simulink model "PID_CARTESIANO"  (R2015a)
settings: Solver=ode45  StartTime=0.0  StopTime=Tfinal  RelTol=1e-3
values from neighbouring files (symbols this model uses):
  Ki1 = 0    [INICIO.m]
  Ki2 = 0    [INICIO.m]
  Ki3 = 0    [INICIO.m]
  Ki4 = 0    [INICIO.m]
  Kp1 = 100    [INICIO.m]
  Kp2 = 100    [INICIO.m]
  Kp3 = 100    [INICIO.m]
  Kp4 = 100    [INICIO.m]
  Kv1 = 10    [INICIO.m]
  Kv2 = 10    [INICIO.m]
  Kv3 = 10    [INICIO.m]
  Kv4 = 10    [INICIO.m]
  Tem = 0.001    [INICIO.m]    (also in circular.m)
undefined symbols (not defined in the file or in its folder): diferencia, mgd, mgi
libraries: simulink x1
settings Model: CovHtmlReporting=off  Creator=ANDRES Y MARCELA  LastModifiedBy=Shadow
settings DataIOCC: SignalLoggingSaveFormat=ModelDataLogs
settings OptimizationCC: ExpressionDepthLimit=2147483647
settings DebuggingCC: UnderspecifiedInitializationDetection=Classic  MergeDetectMultiDrivingBlocksExec=none  SolverPrmCheckMsg=warning  FcnCallInpInsideContextMsg=EnableAllAsWarning  StateNameClashWarn=warning
settings GRTTargetCC: CombineOutputUpdateFcns=off  GRTInterface=on

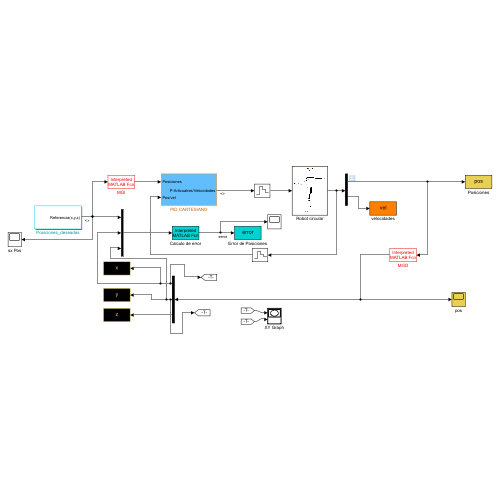
[thumbnail: Simulink's stored preview of the top-level diagram]
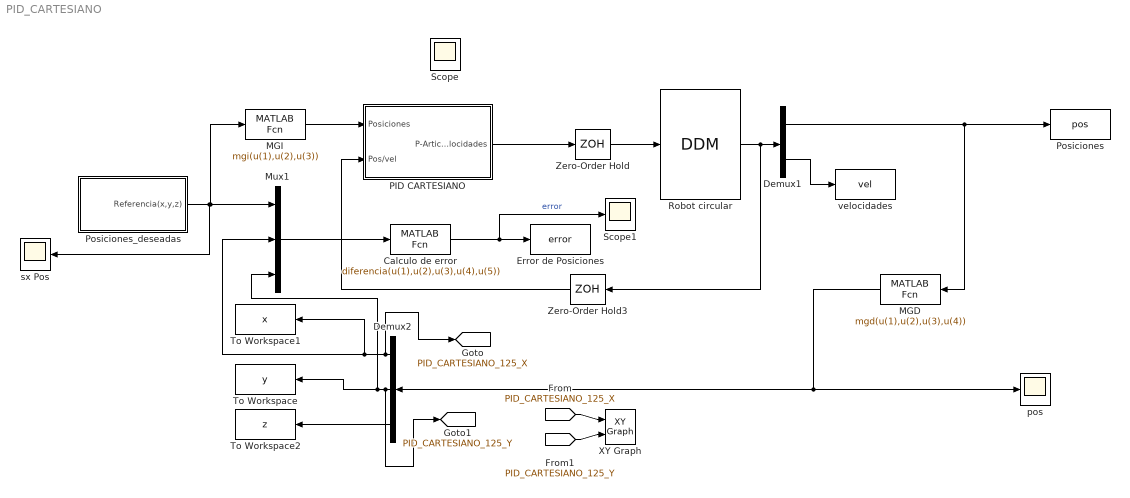
== system PID_CARTESIANO ==
  Calculo de error : MATLABFcn  MATLABFcn=diferencia(u(1),u(2),u(3),u(4),u(5))
  Demux1 : Demux  Outputs=2
  Demux2 : Demux  Outputs=3
  Error de Posiciones : ToWorkspace  VariableName=error  SampleTime=-1
  MGD : MATLABFcn  MATLABFcn=mgd(u(1),u(2),u(3),u(4))
  MGI : MATLABFcn  MATLABFcn=mgi(u(1),u(2),u(3))
  Mux1 : Mux  Inputs=3
  PID CARTESIANO : Subsystem
  Posiciones : ToWorkspace  VariableName=pos  SampleTime=-1
  Posiciones_deseadas : Subsystem
  Robot circular : S-Function  FunctionName=DDM  Parameters=QI  SFunctionDeploymentMode=off  EnableBusSupport=off
      mask Display:
      | %  find_system('Name','robot');
      |  image(imread('robot.jpg'))
  Scope1 : Scope
      settings: TimeRange=auto  MaxDataPoints=5000  SaveToWorkspace=off  SaveName=ScopeData2  YMin=-0.00006  YMax=0.00051  SampleTime=-1
  To Workspace : ToWorkspace  VariableName=y  SampleTime=-1
  To Workspace1 : ToWorkspace  VariableName=x  SampleTime=-1
  To Workspace2 : ToWorkspace  VariableName=z  SampleTime=-1
  XY Graph : simulink/Sinks/XY Graph  xmin=-1  xmax=1  ymin=-1  ymax=1  st=-1
  Zero-Order Hold : ZeroOrderHold  SampleTime=Tem
  Zero-Order Hold3 : ZeroOrderHold  SampleTime=Tem
  pos : Scope
      settings: TimeRange=3  LimitDataPoints=on  MaxDataPoints=5000  SaveToWorkspace=off  SaveName=ScopeData4  YMin=0.36498  YMax=0.51503  SampleTime=-1
  sx Pos : Scope
      settings: TimeRange=3  LimitDataPoints=on  MaxDataPoints=5000  SaveToWorkspace=off  SaveName=ScopeData2  YMin=0.365  YMax=0.515  SampleTime=-1
  velocidades : ToWorkspace  VariableName=vel  SampleTime=-1
  Scope : Scope
      settings: TimeRange=auto  MaxDataPoints=5000  SaveToWorkspace=off  YMin=-1.01882  YMax=0.95883  SampleTime=-1
  tag scope: PID_CARTESIANO_125_X=global, PID_CARTESIANO_125_Y=global
  wires:
  MGI/1 -> PID CARTESIANO/1(Posiciones)
  Demux1/2 -> velocidades/1
  Posiciones_deseadas/1(Referencia(x,y,z)) -> MGI/1, Mux1/1, sx Pos/1
  Demux2/3 -> To Workspace2/1
  Robot circular/1 -> Zero-Order Hold3/1, Demux1/1
  Zero-Order Hold/1 -> Robot circular/1
  Mux1/1 -> Calculo de error/1
  Zero-Order Hold3/1 -> PID CARTESIANO/2(Pos/vel)
  Calculo de error/1 -> Error de Posiciones/1, Scope1/1  "error"
  Demux2/1 -> To Workspace1/1, Mux1/2, [PID_CARTESIANO_125_X]
  Demux2/2 -> To Workspace/1, Mux1/3, [PID_CARTESIANO_125_Y]
  MGD/1 -> pos/1, Demux2/1
  Demux1/1 -> Posiciones/1, MGD/1
  PID CARTESIANO/1(P-Articualres/Velocidades) -> Zero-Order Hold/1
  [PID_CARTESIANO_125_X] -> XY Graph/1
  [PID_CARTESIANO_125_Y] -> XY Graph/2

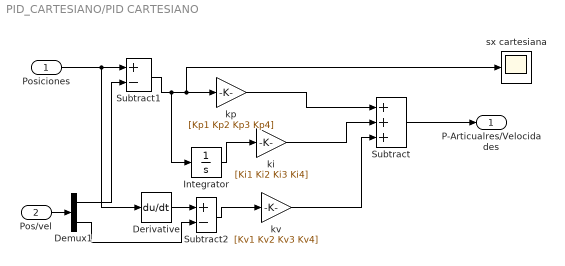
== system PID_CARTESIANO/PID CARTESIANO ==
  Posiciones : Inport
  Pos/vel : Inport  Port=2
  Demux1 : Demux  Outputs=2
  Derivative : Derivative
  Integrator : Integrator
  Subtract : Sum  Inputs=+++
  Subtract1 : Sum  Inputs=+-
  Subtract2 : Sum  Inputs=+-
  ki : Gain  Gain=[Ki1 Ki2 Ki3 Ki4]
  kp : Gain  Gain=[Kp1 Kp2 Kp3 Kp4]
  kv : Gain  Gain=[Kv1 Kv2 Kv3 Kv4]
  sx cartesiana : Scope
      settings: TimeRange=3  LimitDataPoints=on  MaxDataPoints=5000  SaveToWorkspace=off  YMin=-0.00012  YMax=0.00023  SampleTime=-1
  P-Articualres/Velocidades : Outport
  wires:
  Subtract1/1 -> Integrator/1, kp/1, sx cartesiana/1
  Derivative/1 -> Subtract2/1
  Subtract2/1 -> kv/1
  kp/1 -> Subtract/1
  Integrator/1 -> ki/1
  Pos/vel/1 -> Demux1/1
  Posiciones/1 -> Derivative/1, Subtract1/1
  Subtract/1 -> P-Articualres/Velocidades/1
  Demux1/1 -> Subtract1/2
  Demux1/2 -> Subtract2/2
  ki/1 -> Subtract/2
  kv/1 -> Subtract/3

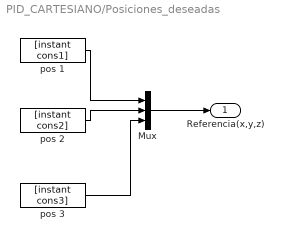
== system PID_CARTESIANO/Posiciones_deseadas ==
  Mux : Mux  Inputs=3
  pos 1 : FromWorkspace  VariableName=[instant cons1]  SampleTime=Tem  ZeroCross=off
  pos 2 : FromWorkspace  VariableName=[instant cons2]  SampleTime=Tem  ZeroCross=off
  pos 3 : FromWorkspace  VariableName=[instant cons3]  SampleTime=Tem  ZeroCross=off
  Referencia(x,y,z) : Outport
  wires:
  pos 1/1 -> Mux/1
  pos 2/1 -> Mux/2
  pos 3/1 -> Mux/3
  Mux/1 -> Referencia(x,y,z)/1
